simulink model "model_wielomianowy"  (R2014b)
settings: Solver=ode45  StartTime=0.0  StopTime=10.0  RelTol=1e-3
values from neighbouring files (symbols this model uses):
  b0 = (x1T-x10)/T    (= 0.1)    [wielomianowy.m]
  c = [b0*T^3/6, -T^2/2; -b0*T^2/2, T]*[xT(2)-xz(2); xT(3)-xz(3)-b0*xz(2)*T]*-12/(b0*T^4)    [wielomianowy.m]
  teta0 = 0    [dynamika.m]    (also in kinematyka.m; monocykl.m = 3; wielomianowy.m)
  x0 = 0    [dynamika.m]    (also in kinematyka.m; monocykl.m = 4; wielomianowy.m = 1)
  x10 = 1    [wielomianowy.m]
  x20 = 2    [wielomianowy.m]
  x30 = 0    [wielomianowy.m]
  y0 = 0    [dynamika.m]    (also in kinematyka.m; monocykl.m = 2; wielomianowy.m = 2)
settings Model: Creator=Dawid Perdek  LastModifiedBy=Dawid Perdek

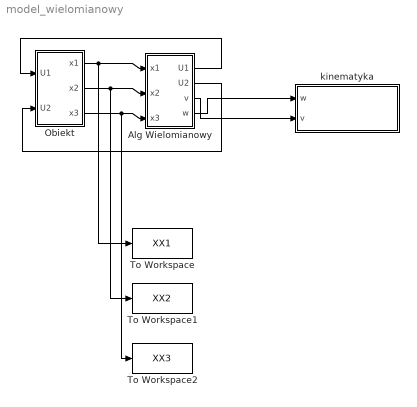
== system model_wielomianowy ==
  Alg Wielomianowy : Subsystem
  Obiekt : Subsystem
  To Workspace : ToWorkspace  VariableName=XX1  SampleTime=-1
  To Workspace1 : ToWorkspace  VariableName=XX2  SampleTime=-1
  To Workspace2 : ToWorkspace  VariableName=XX3  SampleTime=-1
  kinematyka : Subsystem
  wires:
  Obiekt/1(x1) -> To Workspace/1, Alg Wielomianowy/1(x1)
  Obiekt/2(x2) -> To Workspace1/1, Alg Wielomianowy/2(x2)
  Obiekt/3(x3) -> To Workspace2/1, Alg Wielomianowy/3(x3)
  Alg Wielomianowy/2(U2) -> Obiekt/2(U2)
  Alg Wielomianowy/1(U1) -> Obiekt/1(U1)
  Alg Wielomianowy/4(w) -> kinematyka/1(w)
  Alg Wielomianowy/3(v) -> kinematyka/2(v)

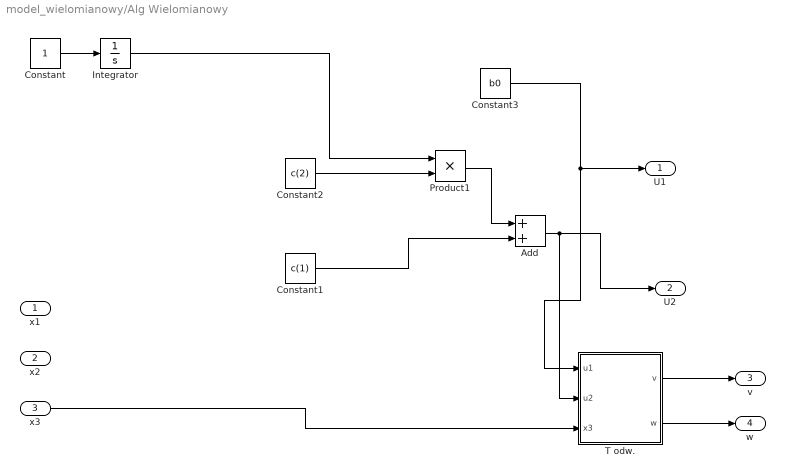
== system model_wielomianowy/Alg Wielomianowy ==
  x1 : Inport
  x2 : Inport  Port=2
  x3 : Inport  Port=3
  Add : Sum
  Constant : Constant
  Constant1 : Constant  Value=c(1)
  Constant2 : Constant  Value=c(2)
  Constant3 : Constant  Value=b0
  Integrator : Integrator
  Product1 : Product
  T odw. : Subsystem
  U1 : Outport
  U2 : Outport  Port=2
  v : Outport  Port=3
  w : Outport  Port=4
  wires:
  Constant/1 -> Integrator/1
  Integrator/1 -> Product1/1
  Constant2/1 -> Product1/2
  Product1/1 -> Add/1
  Constant1/1 -> Add/2
  Add/1 -> T odw./2(u2), U2/1
  Constant3/1 -> T odw./1(u1), U1/1
  x3/1 -> T odw./3(x3)
  T odw./2(w) -> w/1
  T odw./1(v) -> v/1

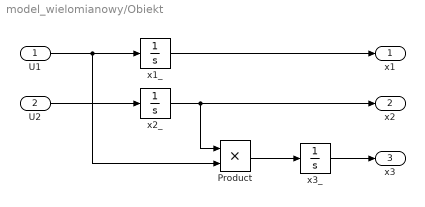
== system model_wielomianowy/Obiekt ==
  U1 : Inport
  U2 : Inport  Port=2
  Product : Product
  x1_ : Integrator  InitialCondition=x10
  x2_ : Integrator  InitialCondition=x20
  x3_ : Integrator  InitialCondition=x30
  x1 : Outport
  x2 : Outport  Port=2
  x3 : Outport  Port=3
  wires:
  U1/1 -> Product/2, x1_/1
  x2_/1 -> x2/1, Product/1
  U2/1 -> x2_/1
  x1_/1 -> x1/1
  x3_/1 -> x3/1
  Product/1 -> x3_/1

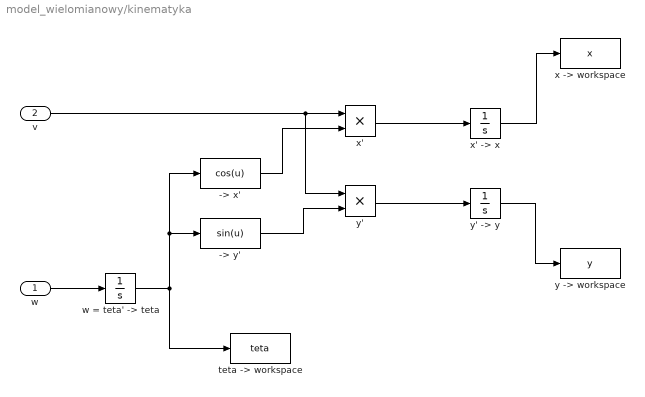
== system model_wielomianowy/kinematyka ==
  w : Inport
  v : Inport  Port=2
  -> x' : Fcn  Expr=cos(u)
  -> y' : Fcn  Expr=sin(u)
  "teta -> workspace" : ToWorkspace  VariableName=teta  SampleTime=-1
  "w = teta' -> teta" : Integrator  InitialCondition=teta0
  "x -> workspace" : ToWorkspace  VariableName=x  SampleTime=-1
  x' : Product
  "x' -> x" : Integrator  InitialCondition=x0
  "y -> workspace" : ToWorkspace  VariableName=y  SampleTime=-1
  y' : Product
  "y' -> y" : Integrator  InitialCondition=y0
  wires:
  w/1 -> "w = teta' -> teta"/1
  v/1 -> y'/1, x'/1
  -> x'/1 -> x'/2
  -> y'/1 -> y'/2
  x'/1 -> "x' -> x"/1
  y'/1 -> "y' -> y"/1
  "x' -> x"/1 -> "x -> workspace"/1
  "y' -> y"/1 -> "y -> workspace"/1
  "w = teta' -> teta"/1 -> "teta -> workspace"/1, -> x'/1, -> y'/1

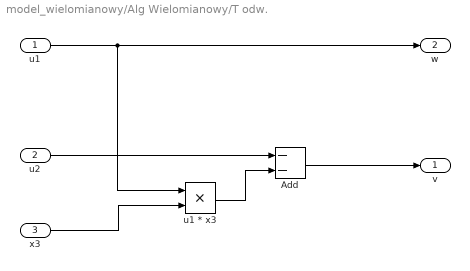
== system model_wielomianowy/Alg Wielomianowy/T odw. ==
  u1 : Inport
  u2 : Inport  Port=2
  x3 : Inport  Port=3
  Add : Sum  Inputs=--
  u1 * x3 : Product
  v : Outport
  w : Outport  Port=2
  wires:
  u1/1 -> w/1, u1 * x3/1
  x3/1 -> u1 * x3/2
  u1 * x3/1 -> Add/2
  u2/1 -> Add/1
  Add/1 -> v/1
